simulink model "slipm3D_zir"  (R2025b)
settings: Solver=ode4  StartTime=0.0  StopTime=t_stop  FixedStep=t_step  RelTol=1e-3
values from neighbouring files (symbols this model uses):
  dx0 = -0.467    [ref_data_zir.m]
  dy0 = 0.467    [ref_data_zir.m]
  t_step = 0.001    [ref_data_zir.m]
  x0 = 0.151    [ref_data_zir.m]
  y0 = 0.05    [ref_data_zir.m]
settings Model: Creator=Admin  LastModifiedBy=Vishal
settings OptimizationCC: ReuseModelBlockBuffer=off
settings RTWCC: GPUComputeCapability=3.5

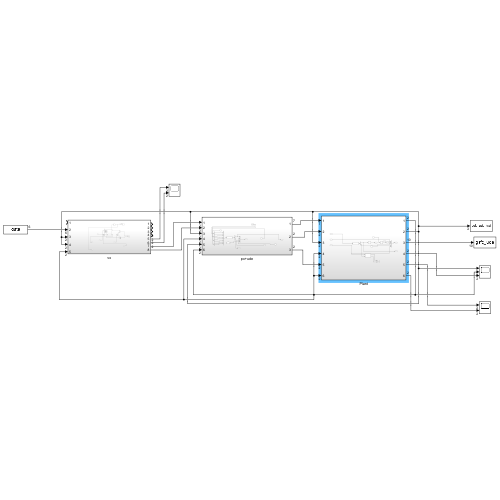
[thumbnail: Simulink's stored preview of the top-level diagram]
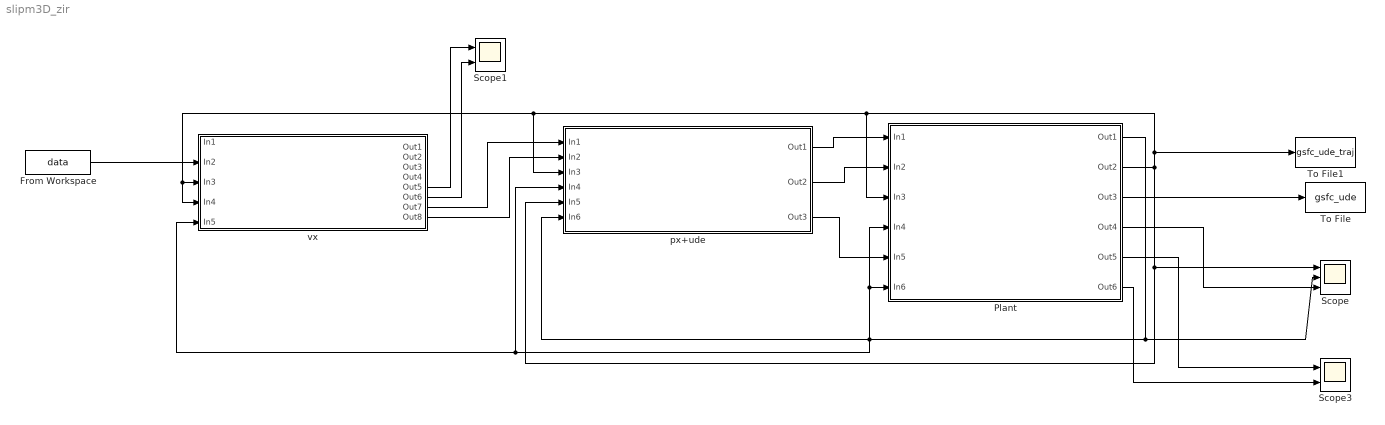
== system slipm3D_zir ==
  From Workspace : FromWorkspace  VariableName=data  OutDataTypeStr=double  SampleTime=t_step
  Plant : Subsystem
  Scope : Scope  NumInputPorts=3
      settings: ActiveDisplayYMinimum=-1  ActiveDisplayYMaximum=1
  Scope1 : Scope  NumInputPorts=2
      settings: ActiveDisplayYMinimum=0.082020223314495683  ActiveDisplayYMaximum=0.48484303163179093
  Scope3 : Scope  NumInputPorts=2
      settings: ActiveDisplayYMinimum=-117.57499094481869  ActiveDisplayYMaximum=124.1749185033682
  To File : ToFile  Filename=gsfc_ude  MatrixName=state_ude
  To File1 : ToFile  Filename=gsfc_ude_traj  MatrixName=sutj
  px+ude : Subsystem
  vx : Subsystem
  wires:
  From Workspace/1 -> vx/2(In2)
  vx/5(Out5) -> Scope1/1
  vx/6(Out6) -> Scope1/2
  vx/7(Out7) -> px+ude/1(In1)
  vx/8(Out8) -> px+ude/2(In2)
  Plant/2(Out2) -> To File1/1, px+ude/3(In3), vx/3(In3), vx/4(In4), Plant/3(In3), px+ude/5(In5), Scope/1
  Plant/1(Out1) -> Plant/6(In6), Plant/4(In4), px+ude/6(In6), vx/5(In5), px+ude/4(In4), Scope/2
  px+ude/1(Out1) -> Plant/1(In1)
  px+ude/2(Out2) -> Plant/2(In2)
  px+ude/3(Out3) -> Plant/5(In5)
  Plant/3(Out3) -> To File/1
  Plant/4(Out4) -> Scope/3
  Plant/5(Out5) -> Scope3/1
  Plant/6(Out6) -> Scope3/2

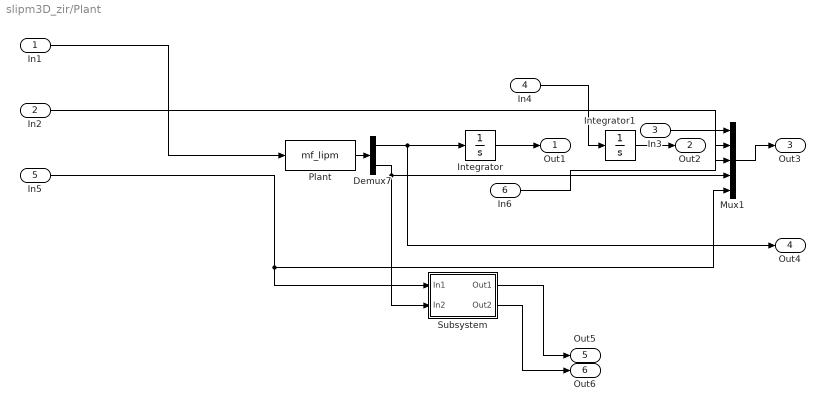
== system slipm3D_zir/Plant ==
  In1 : Inport
  In2 : Inport  Port=2
  In3 : Inport  Port=3
  In4 : Inport  Port=4
  In5 : Inport  Port=5
  In6 : Inport  Port=6
  Demux7 : Demux  Outputs=2
  Integrator : Integrator  InitialCondition=[dx0,dy0]
  Integrator1 : Integrator  InitialCondition=[x0,y0]
  Mux1 : Mux  Inputs=5
  Plant : MATLABFcn  MATLABFcn=mf_lipm  OutputDimensions=4
  Subsystem : Subsystem
  Out1 : Outport
  Out2 : Outport  Port=2
  Out3 : Outport  Port=3
  Out4 : Outport  Port=4
  Out5 : Outport  Port=5
  Out6 : Outport  Port=6
  wires:
  Plant/1 -> Demux7/1
  Subsystem/2(Out2) -> Out6/1
  Demux7/2 -> Subsystem/2(In2), Mux1/4
  Demux7/1 -> Out4/1, Integrator/1
  Mux1/1 -> Out3/1
  Integrator1/1 -> Out2/1
  In5/1 -> Subsystem/1(In1), Mux1/5
  In3/1 -> Mux1/1
  In4/1 -> Integrator1/1
  In6/1 -> Mux1/2
  Integrator/1 -> Out1/1
  Subsystem/1(Out1) -> Out5/1
  In2/1 -> Mux1/3
  In1/1 -> Plant/1

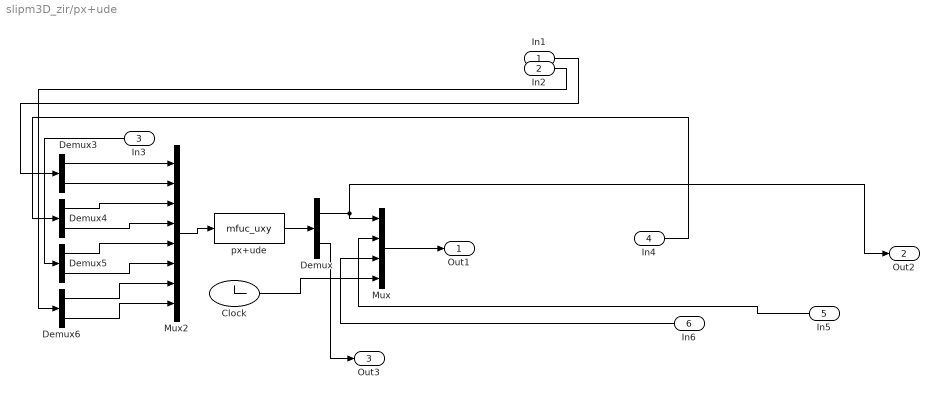
== system slipm3D_zir/px+ude ==
  In1 : Inport
  In2 : Inport  Port=2
  In3 : Inport  Port=3
  In4 : Inport  Port=4
  In5 : Inport  Port=5
  In6 : Inport  Port=6
  Clock : Clock
  Demux{,3..6} (5 alike) : Demux  Outputs=2
  Mux : Mux
  Mux2 : Mux  Inputs=8
  px+ude : MATLABFcn  MATLABFcn=mfuc_uxy  OutputDimensions=4
  Out1 : Outport
  Out2 : Outport  Port=2
  Out3 : Outport  Port=3
  wires:
  Mux2/1 -> px+ude/1
  In1/1 -> Demux3/1
  Demux5/1 -> Mux2/5
  Demux/1 -> Out2/1, Mux/1
  Mux/1 -> Out1/1
  px+ude/1 -> Demux/1
  Demux5/2 -> Mux2/6
  Demux4/2 -> Mux2/4
  Demux3/2 -> Mux2/2
  Demux3/1 -> Mux2/1
  In5/1 -> Mux/2
  Demux4/1 -> Mux2/3
  Clock/1 -> Mux/4
  Demux6/2 -> Mux2/8
  Demux6/1 -> Mux2/7
  In2/1 -> Demux6/1
  In3/1 -> Demux5/1
  Demux/2 -> Out3/1
  In6/1 -> Mux/3
  In4/1 -> Demux4/1

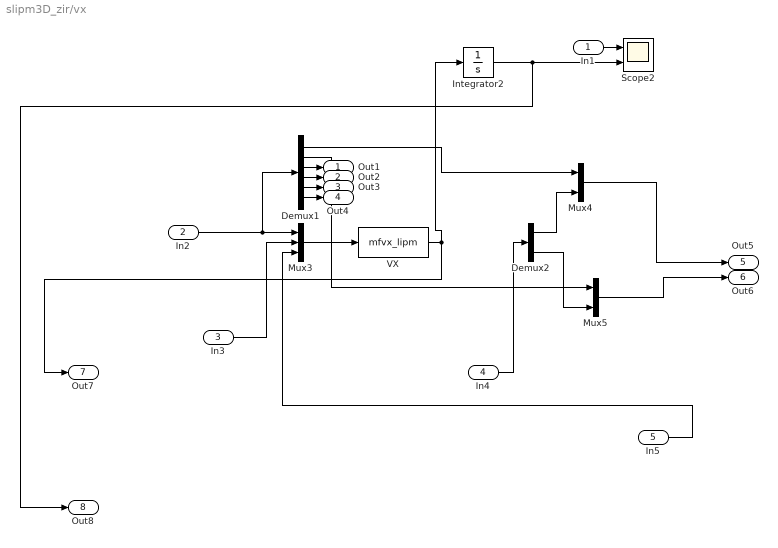
== system slipm3D_zir/vx ==
  In1 : Inport
  In2 : Inport  Port=2
  In3 : Inport  Port=3
  In4 : Inport  Port=4
  In5 : Inport  Port=5
  Demux1 : Demux  Outputs=6
  Demux2 : Demux  Outputs=2
  Integrator2 : Integrator
  Mux3 : Mux  Inputs=3
  Mux4 : Mux  Inputs=2
  Mux5 : Mux  Inputs=2
  Scope2 : Scope  NumInputPorts=2
      settings: ActiveDisplayYMinimum=-1  ActiveDisplayYMaximum=1
  VX : MATLABFcn  MATLABFcn=mfvx_lipm  OutputDimensions=2
  Out1 : Outport
  Out2 : Outport  Port=2
  Out3 : Outport  Port=3
  Out4 : Outport  Port=4
  Out5 : Outport  Port=5
  Out6 : Outport  Port=6
  Out7 : Outport  Port=7
  Out8 : Outport  Port=8
  wires:
  In2/1 -> Demux1/1, Mux3/1
  VX/1 -> Out7/1, Integrator2/1
  Demux2/2 -> Mux5/2
  Mux3/1 -> VX/1
  In1/1 -> Scope2/1
  Demux1/6 -> Out4/1
  Integrator2/1 -> Out8/1, Scope2/2
  Demux2/1 -> Mux4/2
  Demux1/1 -> Mux4/1
  In4/1 -> Demux2/1
  Demux1/2 -> Mux5/1
  Demux1/3 -> Out1/1
  Demux1/4 -> Out2/1
  Demux1/5 -> Out3/1
  Mux5/1 -> Out6/1
  Mux4/1 -> Out5/1
  In5/1 -> Mux3/3
  In3/1 -> Mux3/2

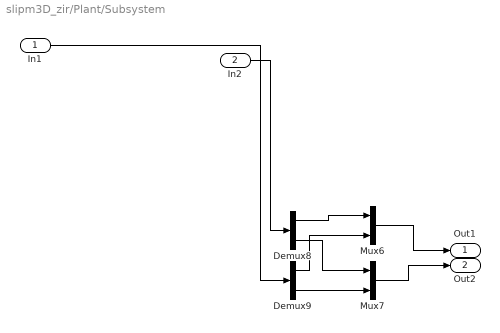
== system slipm3D_zir/Plant/Subsystem ==
  In1 : Inport
  In2 : Inport  Port=2
  Demux8 : Demux  Outputs=2
  Demux9 : Demux  Outputs=2
  Mux6 : Mux  Inputs=2
  Mux7 : Mux  Inputs=2
  Out1 : Outport
  Out2 : Outport  Port=2
  wires:
  Demux9/1 -> Mux6/2
  Demux8/2 -> Mux7/1
  Mux7/1 -> Out2/1
  Demux8/1 -> Mux6/1
  In1/1 -> Demux9/1
  Demux9/2 -> Mux7/2
  In2/1 -> Demux8/1
  Mux6/1 -> Out1/1
